simulink model "StatKarakteristika"  (R2020b)
settings: Solver=VariableStepAuto  StartTime=0.0  StopTime=10.0  RelTol=1e-3
undefined symbols (not defined in the file or in its folder): K
libraries: PoKeysIOInterface x1
settings Model: Creator=64210381  LastModifiedBy=Acer

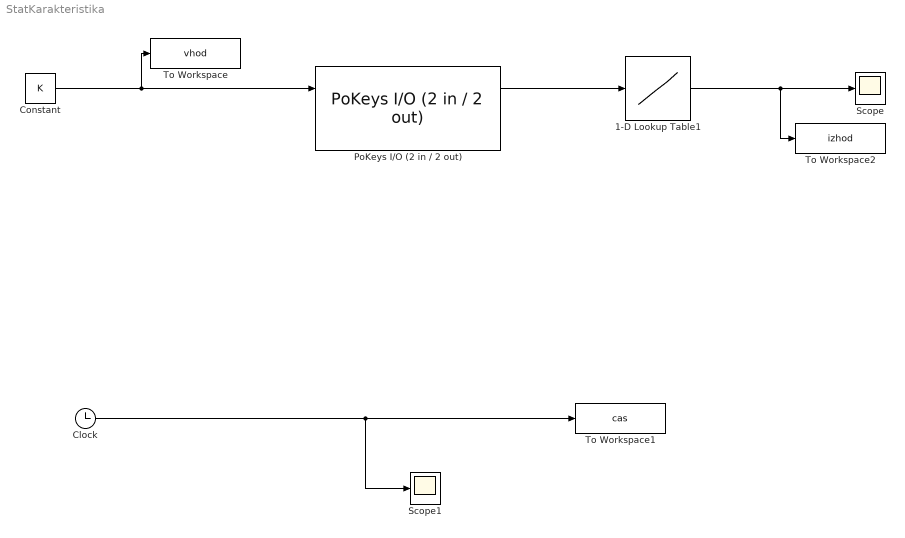
== system StatKarakteristika ==
  1-D Lookup Table1 : Lookup_n-D  NumberOfTableDimensions=1  BreakpointsForDimension1=[0.83, 3.52, 6]  Table=[177, 90, 14]  SampleTime=0.1  InternalRulePriority=Speed  RndMeth=Simplest  InputSameDT=on
  Clock : Clock
  Constant : Constant  Value=K
  PoKeys I/O (2 in / 2 out) : PoKeysIOInterface/PoKeys I//O (2 in // 2 out)  MaxPowerLimit=100.0  IOTs=0.002  IOSerial=507
      settings: SourceProductName=PoKeys I/O interface
  Scope : Scope
  Scope1 : Scope
  To Workspace : ToWorkspace  VariableName=vhod  SampleTime=-1
  To Workspace1 : ToWorkspace  VariableName=cas  SampleTime=-1
  To Workspace2 : ToWorkspace  VariableName=izhod  SampleTime=-1
  wires:
  Constant/1 -> To Workspace/1, PoKeys I/O (2 in / 2 out)/1
  PoKeys I/O (2 in / 2 out)/1 -> 1-D Lookup Table1/1
  Clock/1 -> To Workspace1/1, Scope1/1
  1-D Lookup Table1/1 -> To Workspace2/1, Scope/1
